simulink library "sm_robot_run_4legs_lib"  (R2020b)
settings: Solver=ode45  StartTime=0.0  StopTime=10.0  RelTol=1e-3
undefined symbols (not defined in the file): bw, d2r, Extr_Data_LinkEndHole, ground, J, joint_damping, k2, knee_torque, l1, l2, L_back, m1, m2, N, r2d, T_cg, t_th, t_w, th2, Trq_propulsive, u_th, u_w, X, Y, Z
libraries: sm_lib x25, nesl_utility x14, fl_lib x13, Contact_Forces_Lib x1, ee_lib x1
(part 2 of 2)

== system sm_robot_run_4legs_lib/Leg/Contact Force Model/Planar/Force Law/Capture floor x-position ==
  x : Inport
  Trigger : TriggerPort  VariantControl=Variant
  x0 : Outport  InitialOutput=x0  VectorParamsAs1DForOutWhenUnconnected=off
  wires:
  x/1 -> x0/1

== system sm_robot_run_4legs_lib/Leg/Contact Force Model/Planar/Force Law/Penalty Force ==
  pen : Inport
  vel : Inport  Port=2
  Action Port : ActionPort
  Gain : Gain  Gain=[-ground.stiffness 0 0;0 -ground.stiffness 0;0 0 0]  Multiplication=Matrix(K*u)  SaturateOnIntegerOverflow=on  OutDataTypeStr=Inherit: Same as input  ParamDataTypeStr=Inherit: Same as input
  Gain1 : Gain  Gain=[-ground.damping 0 0;0 -ground.damping 0;0 0 0]  Multiplication=Matrix(K*u)  SaturateOnIntegerOverflow=on  OutDataTypeStr=Inherit: Same as input  ParamDataTypeStr=Inherit: Same as input
  Saturation : Saturate  UpperLimit=[inf inf inf]  LowerLimit=[-inf 0 -inf]
  Sum : Sum  Inputs=|++  SaturateOnIntegerOverflow=on
  force : Outport  InitialOutput=0  VectorParamsAs1DForOutWhenUnconnected=off
  wires:
  pen/1 -> Gain/1
  Gain/1 -> Sum/1
  Sum/1 -> Saturation/1
  Gain1/1 -> Sum/2
  vel/1 -> Gain1/1
  Saturation/1 -> force/1

== system sm_robot_run_4legs_lib/Leg/Contact Force Model/Planar/Force Law/Zero Force ==
  Action Port : ActionPort
  Zero Force : Constant  Value=[0;0;0]
  force : Outport  InitialOutput=0  VectorParamsAs1DForOutWhenUnconnected=off
  wires:
  Zero Force/1 -> force/1

== system sm_robot_run_4legs_lib/Leg/Knee Actuator/Torque for knee retraction/Enabled Subsystem/Angle profile ==
  time : Inport
  Constant angle t >= 6*T_cg/4 : Constant  Value=0
  Gain : Gain  Gain=-1
  Half sine wave 0 < t < 6*T_cg/4 : Subsystem
  Switch : Switch  Threshold=6*T_cg/4
      settings: AttributesFormatString=Threshold = %<Threshold>
  y : Outport  VectorParamsAs1DForOutWhenUnconnected=off
  wires:
  Gain/1 -> y/1
  time/1 -> Half sine wave 0 < t < 6*T_cg/4/1(time), Switch/2
  Half sine wave 0 < t < 6*T_cg/4/1(y) -> Switch/3
  Constant angle t >= 6*T_cg/4/1 -> Switch/1
  Switch/1 -> Gain/1

== system sm_robot_run_4legs_lib/Leg/Knee Actuator/Torque for knee retraction/Enabled Subsystem/Angle profile/Half sine wave 0 < t < 6*T_cg//4 ==
  time : Inport
  A : Gain  Gain=50
  Constant2 : Constant  Value=th2*r2d*0
  Sum : Sum  Inputs=++|
  sin(wt) : Trigonometry
  w : Gain  Gain=2*pi/(3*T_cg)
  y : Outport  VectorParamsAs1DForOutWhenUnconnected=off
  wires:
  time/1 -> w/1
  Sum/1 -> y/1
  Constant2/1 -> Sum/1
  A/1 -> Sum/2
  sin(wt)/1 -> A/1
  w/1 -> sin(wt)/1
